simulink library "thc"  (R2021b)
settings: Solver=VariableStepAuto  StartTime=0.0  StopTime=10.0  RelTol=1e-3
undefined symbols (not defined in the file or in its folder): ATHC_APTCQA_X_C, ATHC_APTCQB_X_C, ATHC_dAy_X_C, ATHC_Qeq_X_kmh, ATHC_VbaseC_X_C, ATHC_VbaseC_Y_W, ATHC_VbaseD_X_C, ATHC_VbaseH_X_C, FALSE, KTHC_ACMaxMinT_sec, KTHC_aDeice_K, KTHC_AGSDefLv_K, KTHC_AGSLv1_K, KTHC_AGSLv2_K, KTHC_AGSLv3_K, KTHC_AGSLv4_K, KTHC_AGSLv5_K, KTHC_AirIntUpdateT_sec, KTHC_APTCOneZoneMax_W, KTHC_APTCPeriod_cnt, KTHC_APTCPWMEN_flg, KTHC_APTCQMaxC_W, KTHC_APTCQminC_W, KTHC_APTCQminD_W, KTHC_APTCQminRe1_W, KTHC_APTCQminRe_W, KTHC_APTCQoffT_cnt, KTHC_APTCQonT_cnt, KTHC_APTCRiLeMaxDff_W, KTHC_APTCRiLeMinDff_W, KTHC_BatInTempDef_C, KTHC_bDeice_K, KTHC_CompMaxDeice_rpm, KTHC_CompMinDeice_rpm, KTHC_CompSotxvOp_K, KTHC_CompSotxvOpLow_rpm, KTHC_CompSpdmax_rpm, KTHC_CompSpdmaxBC1_rpm, KTHC_CompSpdmaxBC_rpm, KTHC_CompSpdmid1_rpm, KTHC_CompSpdmid2_rpm, KTHC_CompSpdmid3_rpm, KTHC_CompSpdmid_rpm, KTHC_CompSpdmin_rpm, KTHC_DAPTCQ1_W, KTHC_DAPTCQ2_W, KTHC_DAPTCQ3_W, KTHC_DcChSetTemp_C, KTHC_DehumidityEN_flg, KTHC_DeiceCycTime_K, KTHC_DriveLevelWPTCBAH1_W, KTHC_DriveLevelWPTCBAH2_W, KTHC_DriveLevelWPTCBAH3_W, KTHC_DriveLevelWPTCBAH4_W, KTHC_DriveT1MinBAH_C, KTHC_DriveT2MaxBAH_C, KTHC_DriveT2MinBAH_C, KTHC_DriveT3MaxBAH_C, KTHC_DriveT3MinBAH_C, KTHC_DriveT4MaxBAH_C ... (+372)
libraries: simulink x140
(part 1 of 10)
settings Model: Creator=FVT20341  LastModifiedBy=FVT22063

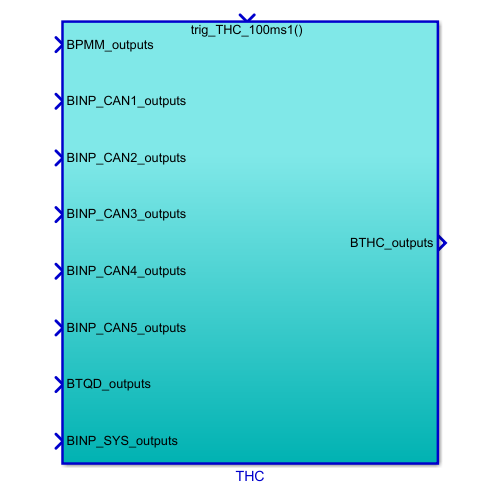
[thumbnail: Simulink's stored preview of the top-level diagram]
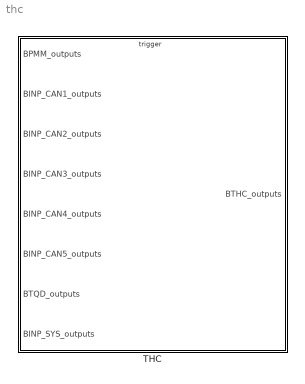
== system thc ==
  THC : Subsystem  TreatAsAtomicUnit=on
      settings: RTWSystemCode=Nonreusable function  RTWFcnNameOpts=Use subsystem name  RTWFileNameOpts=Use subsystem name

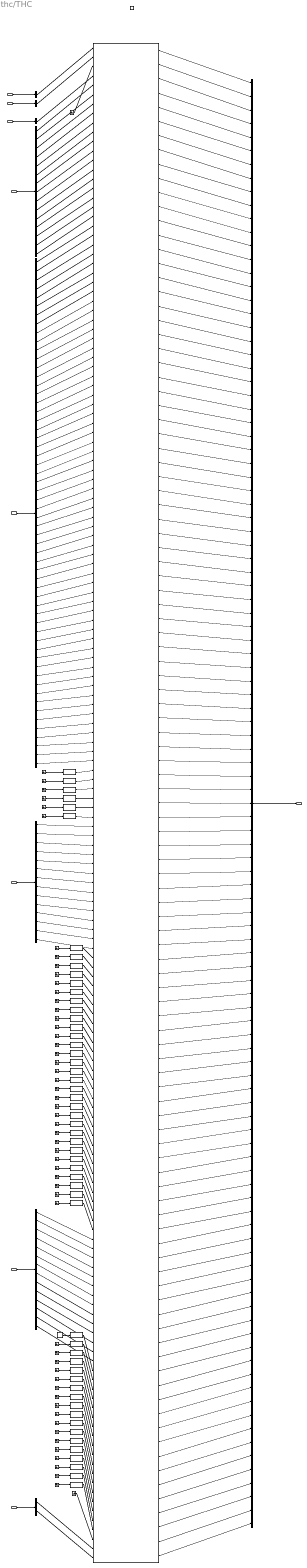
== system thc/THC ==
  BPMM_outputs : Inport  OutDataTypeStr=Bus: BPMM_outputs
  BINP_CAN1_outputs : Inport  Port=2  OutDataTypeStr=Bus: BINP_CAN1_outputs
  BINP_CAN2_outputs : Inport  Port=3  OutDataTypeStr=Bus: BINP_CAN2_outputs
  BINP_CAN3_outputs : Inport  Port=4  OutDataTypeStr=Bus: BINP_CAN3_outputs
  BINP_CAN4_outputs : Inport  Port=5  OutDataTypeStr=Bus: BINP_CAN4_outputs
  BINP_CAN5_outputs : Inport  Port=6  OutDataTypeStr=Bus: BINP_CAN5_outputs
  BTQD_outputs : Inport  Port=7  OutDataTypeStr=Bus: BTQD_outputs
  BINP_SYS_outputs : Inport  Port=8  OutDataTypeStr=Bus: BINP_SYS_outputs
  trig_THC_100ms1 : TriggerPort  TriggerType=function-call  VariantControl=(inherit)
  Bus Creator : BusCreator  Inputs=107  OutDataTypeStr=Bus: BTHC_outputs  NonVirtualBus=on
  Bus Selector : BusSelector  OutputSignals=VINP_FlashACModeMem_enum,VINP_FlashFace_flg,VINP_FlashFoot_flg,VINP_FlashFrost_flg,VINP_FlashFaceM_flg,VINP_FlashFootM_flg,VINP_FlashCCUSyncSts_flg,VINP_FlashACForceOFF_flg,VINP_FlashsigRecircSt_flg,VINP_FlashRecAutoFlg_flg,VINP_FlashAirIntenZone1M_enum,VINP_Flashfdefog_flg,VINP_FlashsigSetTempZon1St_C,VINP_FlashsigSetTempZon2StM_C
  Bus Selector1 : BusSelector  OutputSignals=VINP_VehSpeed_kph
  Bus Selector2 : BusSelector  OutputSignals=VINP_HVBMTempMax_C,VINP_HVBMTempMin_C,VINP_OBCTemp_C,VINP_DCDCTemp_C,VINP_RrTMTemp_C,VINP_RrMCUTemp_C,VINP_FrTMTemp_C,VINP_FrMCUTemp_C,VINP_ChrgPlugSta_enum,VINP_FrLLCTemp_C,VINP_RrLLCTemp_C,VINP_HVBIsoImpedenceN_Megaohm,VINP_HVBIsoImpedenceP_Megaohm,VINP_HVBHVILErr_flg,VINP_HVBattSOC_pct
  Bus Selector3 : BusSelector  OutputSignals=VINP_PTHighTact_C,VINP_COMPStatorSpd_rpm,VINP_CompProEN_flg,VINP_PTLowP1_KPa,VINP_PTLowT1_C,VINP_PTLowP2_KPa,VINP_PTLowT2_C,VINP_PTHighP_KPa,VINP_Tamb_C,VINP_BatInTemp_C,VINP_BatOutTemp_C,VINP_MotorInTemp_C,VINP_MotorOutTemp_C,VINP_Tincar_C,VINP_SolarL_W,VINP_SolarR_W,VINP_Tevap_C,VINP_TFaceL_C,VINP_TFaceR_C,VINP_TFootL_C,VINP_TFootR_C,VINP_TFootRr_C,VINP_TFaceRr_C,VINP_EACProtectEnable_enum,VINP_TambErr_enum,VINP_SolarLErr_enum,VINP_SolarRErr_enum,VINP_TevapErr_enum,VINP_TFaceLErr_enum,VINP_TFaceRErr_enum,VINP_TFootLErr_enum,VINP_TFootRErr_enum,VINP_TFaceRrErr_enum,VINP_TFootRrErr_enum,VINP_TincarErr_enum,VINP_BatInTempErr_enum,VINP_MotorInTempErr_enum,VINP_MotorOutTempErr_enum,VINP_FanErr_enum,VINP_AGSErr_enum,VINP_EWP3Err_enum,VINP_PTHighPErr_enum,VINP_PTHighTactErr_enum,VINP_SOV1Err_enum,VINP_SOV2Err_enum,VINP_SOV3Err_enum,VINP_EXV1Err_enum,VINP_EXV2Err_enum,VINP_COMPErr_enum,VINP_BlowerErr_enum,VINP_PTLowP1Err_enum,VINP_PTLowT1Err_enum,VINP_PTLowP2Err_enum,VINP_PTLowT2Err_enum,VINP_SOTXVErr_enum,VINP_FrntPTCRearLeActHeatPwr_W,VINP_FrntPTCRearRiActHeatPwr_W,VINP_FrntPTCRiActHeatPwr_W
  Bus Selector4 : BusSelector  OutputSignals=VINP_OFFACMODE_enum,VINP_FCPFrEvtBtnACMaxReq_flg,VINP_FCPFrEvtBtnACReq_flg,VINP_FCPFrEvtBtnAutoReq_flg,VINP_FCPFrEvtBtnSyncReq_flg,VINP_sigAirIntenZon1Req_enum,VINP_sigRecircReq_flg,VINP_sigFaceReq_flg,VINP_sigFootReq_flg,VINP_sigDfrstReq_flg,VINP_sigSetTempZon1Req_C,VINP_CANMsgValidIVI2_flg,VINP_sigSetTempZon2Req_C,VINP_SmartEcoModeSW_flg
  Bus Selector5 : BusSelector  OutputSignals=VTQD_ShiftGearPosn_enum
  Bus Selector6 : BusSelector  OutputSignals=VINP_RemoteACTemp_C,VINP_RemoteAutoReq_flg
  Bus Selector7 : BusSelector  OutputSignals=VPMM_PowerSta_enum
  Constant : Constant  Value=4
  Data Type Conversion{,1..4,6,8,10,12..35,48..50} (35 alike) : DataTypeConversion  OutDataTypeStr=uint8
  Data Type Conversion{5,7,9,11,36..47,55..57} (19 alike) : DataTypeConversion  OutDataTypeStr=boolean
  Ground{,1..19,25..26,28,37..54,56,58..70} (55 alike) : Ground
  ThermalControl : Subsystem
  BTHC_outputs : Outport  OutDataTypeStr=Bus: BTHC_outputs
  wires:
  BPMM_outputs/1 -> Bus Selector7/1
  Bus Selector7/1 -> ThermalControl/1(VPMM_PwrSta_enum)  "<VPMM_PowerSta_enum>"
  BINP_CAN1_outputs/1 -> Bus Selector1/1
  Bus Selector1/1 -> ThermalControl/4(VINP_VehSpeed_kph)  "<VINP_VehSpeed_kph>"
  BINP_CAN3_outputs/1 -> Bus Selector2/1
  Bus Selector2/3 -> ThermalControl/7(VINP_OBCTemp_C)  "<VINP_OBCTemp_C>"
  Bus Selector2/4 -> ThermalControl/8(VINP_DCDCTemp_C)  "<VINP_DCDCTemp_C>"
  Bus Selector2/2 -> ThermalControl/6(VINP_HVBMTempMin_C)  "<VINP_HVBMTempMin_C>"
  Bus Selector2/5 -> ThermalControl/9(VINP_RrTMTemp_C)  "<VINP_RrTMTemp_C>"
  Bus Selector2/1 -> ThermalControl/5(VINP_HVBMTempMax_C)  "<VINP_HVBMTempMax_C>"
  Bus Selector2/6 -> ThermalControl/10(VINP_RrMCUTemp_C)  "<VINP_RrMCUTemp_C>"
  Bus Selector2/7 -> ThermalControl/11(VINP_FrTMTemp_C)  "<VINP_FrTMTemp_C>"
  Bus Selector2/8 -> ThermalControl/12(VINP_FrMCUTemp_C)  "<VINP_FrMCUTemp_C>"
  ThermalControl/32(VTHC_sigClntTHvBattOut_C) -> Bus Creator/32  "VTHC_sigClntTHvBattOut_C"
  ThermalControl/31(VTHC_sigSetTempZon2St_C) -> Bus Creator/31  "VTHC_sigSetTempZon2St_C"
  ThermalControl/30(VTHC_sigSetTempZon1St_C) -> Bus Creator/30  "VTHC_sigSetTempZon1St_C"
  ThermalControl/29(VTHC_sigRecircSt_flg) -> Bus Creator/29  "VTHC_sigRecircSt_flg"
  ThermalControl/28(VTHC_sigWindDirZon1St_enum) -> Bus Creator/28  "VTHC_sigWindDirZon1St_enum"
  ThermalControl/27(VTHC_sigAirIntenZon1St_enum) -> Bus Creator/27  "VTHC_sigAirIntenZon1St_enum"
  ThermalControl/26(VTHC_CCUSyncLampSts_flg) -> Bus Creator/26  "VTHC_CCUSyncLampSts_flg"
  ThermalControl/25(VTHC_CCUACMaxLampSts_flg) -> Bus Creator/25  "VTHC_CCUACMaxLampSts_flg"
  ThermalControl/24(VTHC_CCUAutoLampSts_flg) -> Bus Creator/24  "VTHC_CCUAutoLampSts_flg"
  ThermalControl/23(VTHC_CCUACLampSts_flg) -> Bus Creator/23  "VTHC_CCUACLampSts_flg"
  ThermalControl/22(VTHC_CabinMode_enum) -> Bus Creator/22  "VTHC_CabinMode_enum"
  ThermalControl/21(VTHC_EDriveMode_enum) -> Bus Creator/21  "VTHC_EDriveMode_enum"
  ThermalControl/20(VTHC_BatteryMode_enum) -> Bus Creator/20  "VTHC_BatteryMode_enum"
  ThermalControl/19(VTHC_FDBlowerCmd_pct) -> Bus Creator/19  "VTHC_FDBlowerCmd_pct"
  ThermalControl/17(VTHC_FDFrRiAPTCHeatPwrCmd_W) -> Bus Creator/17  "VTHC_FDFrRiAPTCHeatPwrCmd_W"
  ThermalControl/18(VTHC_FDRrAPTCHeatPwrCmd_W) -> Bus Creator/18  "VTHC_FDRrAPTCHeatPwrCmd_W"
  ThermalControl/16(VTHC_FDFrLeAPTCHeatPwrCmd_W) -> Bus Creator/16  "VTHC_FDFrLeAPTCHeatPwrCmd_W"
  ThermalControl/15(VTHC_FDEWP3Cmd_enum) -> Bus Creator/15  "VTHC_FDEWP3Cmd_enum"
  ThermalControl/14(VTHC_FDEWP2Cmd_enum) -> Bus Creator/14  "VTHC_FDEWP2Cmd_enum"
  ThermalControl/13(VTHC_FDEWP1Cmd_enum) -> Bus Creator/13  "VTHC_FDEWP1Cmd_enum"
  ThermalControl/12(VTHC_FDAGSCmd_enum) -> Bus Creator/12  "VTHC_FDAGSCmd_enum"
  ThermalControl/11(VTHC_CoolgFanActDuty_pct) -> Bus Creator/11  "VTHC_CoolgFanActDuty_pct"
  ThermalControl/10(VTHC_FDFrWPTCHeatPwrCmd_W) -> Bus Creator/10  "VTHC_FDFrWPTCHeatPwrCmd_W"
  ThermalControl/9(VTHC_FDTWVCmd_pct) -> Bus Creator/9  "VTHC_FDTWVCmd_pct"
  ThermalControl/8(VTHC_FDFWVCmd_flg) -> Bus Creator/8  "VTHC_FDFWVCmd_flg"
  ThermalControl/7(VTHC_FDSOTXVCmd_flg) -> Bus Creator/7  "VTHC_FDSOTXVCmd_flg"
  ThermalControl/6(VTHC_FDEXV2Cmd_step) -> Bus Creator/6  "VTHC_FDEXV2Cmd_step"
  ThermalControl/5(VTHC_FDEXV1Cmd_step) -> Bus Creator/5  "VTHC_FDEXV1Cmd_step"
  ThermalControl/4(VTHC_FDSOV3Cmd_flg) -> Bus Creator/4  "VTHC_FDSOV3Cmd_flg"
  ThermalControl/3(VTHC_FDSOV2Cmd_flg) -> Bus Creator/3  "VTHC_FDSOV2Cmd_flg"
  ThermalControl/2(VTHC_FDSOV1Cmd_flg) -> Bus Creator/2  "VTHC_FDSOV1Cmd_flg"
  ThermalControl/1(VTHC_FDCompCmd_rpm) -> Bus Creator/1  "VTHC_FDCompCmd_rpm"
  Bus Creator/1 -> BTHC_outputs/1  "BTHC_outputs"
  BINP_CAN4_outputs/1 -> Bus Selector3/1  "BINP_CAN4_outputs"
  Bus Selector3/4 -> ThermalControl/23(VINP_PTLowP1_kPa)  "<VINP_PTLowP1_KPa>"
  Bus Selector3/5 -> ThermalControl/24(VINP_PTLowT1_C)  "<VINP_PTLowT1_C>"
  Bus Selector3/6 -> ThermalControl/25(VINP_PTLowP2_kPa)  "<VINP_PTLowP2_KPa>"
  Bus Selector3/7 -> ThermalControl/26(VINP_PTLowT2_C)  "<VINP_PTLowT2_C>"
  Bus Selector3/8 -> ThermalControl/27(VINP_PTHighP_kPa)  "<VINP_PTHighP_KPa>"
  Bus Selector3/9 -> ThermalControl/28(VINP_Tamb_C)  "<VINP_Tamb_C>"
  Bus Selector3/10 -> ThermalControl/29(VINP_BatInTemp_C)  "<VINP_BatInTemp_C>"
  Bus Selector3/11 -> ThermalControl/30(VINP_BatOutTemp_C)  "<VINP_BatOutTemp_C>"
  Bus Selector3/12 -> ThermalControl/31(VINP_MotorInTemp_C)  "<VINP_MotorInTemp_C>"
  Bus Selector3/13 -> ThermalControl/32(VINP_MotorOutTemp_C)  "<VINP_MotorOutTemp_C>"
  Bus Selector3/14 -> ThermalControl/33(VINP_Tincar_C)  "<VINP_Tincar_C>"
  Bus Selector3/15 -> ThermalControl/34(VINP_SolarL_W)  "<VINP_SolarL_W>"
  Bus Selector3/16 -> ThermalControl/35(VINP_SolarR_W)  "<VINP_SolarR_W>"
  Bus Selector3/17 -> ThermalControl/36(VINP_Tevap_C)  "<VINP_Tevap_C>"
  Bus Selector3/18 -> ThermalControl/37(VINP_TFaceL_C)  "<VINP_TFaceL_C>"
  Bus Selector3/19 -> ThermalControl/38(VINP_TFaceR_C)  "<VINP_TFaceR_C>"
  Bus Selector3/20 -> ThermalControl/39(VINP_TFootL_C)  "<VINP_TFootL_C>"
  Bus Selector3/21 -> ThermalControl/40(VINP_TFootR_C)  "<VINP_TFootR_C>"
  Bus Selector3/22 -> ThermalControl/41(VINP_TFootRr_C)  "<VINP_TFootRr_C>"
  Bus Selector3/23 -> ThermalControl/42(VINP_TFaceRr_C)  "<VINP_TFaceRr_C>"
  BINP_CAN2_outputs/1 -> Bus Selector4/1  "BINP_CAN2_outputs"
  Bus Selector4/2 -> ThermalControl/85(VINP_FCPFrEvtBtnACMaxReq_flg)  "<VINP_FCPFrEvtBtnACMaxReq_flg>"
  Bus Selector4/3 -> ThermalControl/86(VINP_FCPFrEvtBtnACReq_flg)  "<VINP_FCPFrEvtBtnACReq_flg>"
  Bus Selector4/4 -> ThermalControl/87(VINP_FCPFrEvtBtnAutoReq_flg)  "<VINP_FCPFrEvtBtnAutoReq_flg>"
  Bus Selector4/5 -> ThermalControl/88(VINP_FCPFrEvtBtnSyncReq_flg)  "<VINP_FCPFrEvtBtnSyncReq_flg>"
  Bus Selector4/6 -> ThermalControl/89(VINP_sigAirIntenZon1Req_enum)  "<VINP_sigAirIntenZon1Req_enum>"
  Bus Selector4/7 -> ThermalControl/90(VINP_sigRecircReq_flg)  "<VINP_sigRecircReq_flg>"
  Bus Selector4/8 -> ThermalControl/91(VINP_sigFaceReq_flg)  "<VINP_sigFaceReq_flg>"
  Bus Selector4/9 -> ThermalControl/92(VINP_sigFootReq_flg)  "<VINP_sigFootReq_flg>"
  Bus Selector4/10 -> ThermalControl/93(VINP_sigFrostReq_flg)  "<VINP_sigDfrstReq_flg>"
  Bus Selector4/11 -> ThermalControl/94(VINP_sigSetTempZon1Req_C)  "<VINP_sigSetTempZon1Req_C>"
  Bus Selector4/12 -> ThermalControl/95(VINP_CANMsgValidIVI2_flg)  "<VINP_CANMsgValidIVI2_flg>"
  Bus Selector4/13 -> ThermalControl/96(VINP_sigSetTempZon2Req_C)  "<VINP_sigSetTempZon2Req_C>"
  Bus Selector2/9 -> ThermalControl/13(VINP_ChrgPlugSta_enum)  "<VINP_ChrgPlugSta_enum>"
  Bus Selector3/2 -> ThermalControl/21(VINP_COMP_StatorSpd_RPM)  "<VINP_COMPStatorSpd_rpm>"
  Bus Selector3/3 -> ThermalControl/22(VINP_CompProEN_flg)  "<VINP_CompProEN_flg>"
  ThermalControl/33(VTHC_sigCbnSolarLeft_W) -> Bus Creator/33  "VTHC_sigCbnSolarLeft_W"
  ThermalControl/34(VTHC_sigClntTHvBattIn_C) -> Bus Creator/34  "VTHC_sigClntTHvBattIn_C"
  ThermalControl/35(VTHC_sigCbnSolarRight_W) -> Bus Creator/35  "VTHC_sigCbnSolarRight_W"
  ThermalControl/36(VTHC_sigAmbAirT_C) -> Bus Creator/36  "VTHC_sigAmbAirT_C"
  ThermalControl/37(VTHC_sigCbnAirT_C) -> Bus Creator/37  "VTHC_sigCbnAirT_C"
  ThermalControl/38(VTHC_ACSubMode_enum) -> Bus Creator/38  "VTHC_ACSubMode_enum"
  ThermalControl/40(VTHC_CompP_K) -> Bus Creator/40  "VTHC_CompP_K"
  ThermalControl/41(VTHC_CompI_K) -> Bus Creator/41  "VTHC_CompI_K"
  ThermalControl/42(VTHC_CompU_K) -> Bus Creator/42  "VTHC_CompU_K"
  ThermalControl/43(VTHC_CompDeltaU_K) -> Bus Creator/43  "VTHC_CompDeltaU_K"
  ThermalControl/44(VTHC_Compe_K) -> Bus Creator/44  "VTHC_Compe_K"
  ThermalControl/45(VTHC_Blowere_K) -> Bus Creator/45  "VTHC_Blowere_K"
  ThermalControl/46(VTHC_BlowerP_K) -> Bus Creator/46  "VTHC_BlowerP_K"
  ThermalControl/47(VTHC_BlowerU_K) -> Bus Creator/47  "VTHC_BlowerU_K"
  ThermalControl/48(VTHC_Vbase_pct) -> Bus Creator/48  "VTHC_Vbase_pct"
  ThermalControl/49(VTHC_BlowerI_K) -> Bus Creator/49  "VTHC_BlowerI_K"
  ThermalControl/50(VTHC_EXV2P_K) -> Bus Creator/50  "VTHC_EXV2P_K"
  ThermalControl/51(VTHC_EXV2I_K) -> Bus Creator/51  "VTHC_EXV2I_K"
  ThermalControl/52(VTHC_EXV2U_K) -> Bus Creator/52  "VTHC_EXV2U_K"
  ThermalControl/53(VTHC_EXV2e_K) -> Bus Creator/53  "VTHC_EXV2e_K"
  ThermalControl/54(VTHC_APTCP_K) -> Bus Creator/54  "VTHC_APTCP_K"
  ThermalControl/55(VTHC_APTCI_K) -> Bus Creator/55  "VTHC_APTCI_K"
  ThermalControl/56(VTHC_APTCU_K) -> Bus Creator/56  "VTHC_APTCU_K"
  ThermalControl/57(VTHC_APTCe_K) -> Bus Creator/57  "VTHC_APTCe_K"
  ThermalControl/58(VTHC_EXV1P_K) -> Bus Creator/58  "VTHC_EXV1P_K"
  ThermalControl/59(VTHC_EXV1I_K) -> Bus Creator/59  "VTHC_EXV1I_K"
  ThermalControl/60(VTHC_EXV1U_K) -> Bus Creator/60  "VTHC_EXV1U_K"
  ThermalControl/61(VTHC_EXV1e_K) -> Bus Creator/61  "VTHC_EXV1e_K"
  BTQD_outputs/1 -> Bus Selector5/1
  Bus Selector5/1 -> ThermalControl/2(VTQD_ShiftGearPosn_enum)  "<VTQD_ShiftGearPosn_enum>"
  Bus Selector3/1 -> ThermalControl/20(VINP_PTHighTact_C)  "<VINP_PTHighTact_C>"
  Bus Selector2/10 -> ThermalControl/14(VINP_FrLLCTemp_C)  "<VINP_FrLLCTemp_C>"
  Bus Selector2/11 -> ThermalControl/15(VINP_RrLLCTemp_C)  "<VINP_RrLLCTemp_C>"
  Ground/1 -> ThermalControl/3(VSCP_AGSCloseSta_flg)
  Bus Selector4/1 -> ThermalControl/84(VINP_OFFACMODE_enum)  "<VINP_OFFACMODE_enum>"
  ThermalControl/39(VTHC_FDRecyAutoCmd_enum) -> Bus Creator/39  "VTHC_FDRecyAutoCmd_enum"
  Bus Selector3/24 -> ThermalControl/43(VINP_EACProtectEnable_enum)  "<VINP_EACProtectEnable_enum>"
  Bus Selector3/25 -> ThermalControl/44(Tamb_Err)  "<VINP_TambErr_enum>"
  Bus Selector3/26 -> ThermalControl/45(SolarL_Err)  "<VINP_SolarLErr_enum>"
  Bus Selector3/27 -> ThermalControl/46(SolarR_Err)  "<VINP_SolarRErr_enum>"
  Bus Selector3/28 -> ThermalControl/47(Tevap_Err)  "<VINP_TevapErr_enum>"
  Bus Selector3/29 -> ThermalControl/48(T_Face_L_Err)  "<VINP_TFaceLErr_enum>"
  Bus Selector3/30 -> ThermalControl/49(T_Face_R_Err)  "<VINP_TFaceRErr_enum>"
  Bus Selector3/31 -> ThermalControl/50(T_Foot_L_Err)  "<VINP_TFootLErr_enum>"
  Bus Selector3/32 -> ThermalControl/51(T_Foot_R_Err)  "<VINP_TFootRErr_enum>"
  Bus Selector3/33 -> ThermalControl/52(T_Face_Rr_Err)  "<VINP_TFaceRrErr_enum>"
  Bus Selector3/34 -> ThermalControl/53(T_Foot_Rr_Err)  "<VINP_TFootRrErr_enum>"
  Bus Selector3/35 -> ThermalControl/54(Tincar_Err)  "<VINP_TincarErr_enum>"
  Bus Selector3/36 -> ThermalControl/55(Bat_In_Temp_Err)  "<VINP_BatInTempErr_enum>"
  Bus Selector3/37 -> ThermalControl/56(Motor_In_Temp_Err)  "<VINP_MotorInTempErr_enum>"
  Bus Selector3/38 -> ThermalControl/57(Motor_Out_Temp_Err)  "<VINP_MotorOutTempErr_enum>"
  Bus Selector3/39 -> ThermalControl/58(Fan_Err)  "<VINP_FanErr_enum>"
  Bus Selector3/40 -> ThermalControl/59(AGS_Err)  "<VINP_AGSErr_enum>"
  Bus Selector3/41 -> ThermalControl/60(EWP3_Err)  "<VINP_EWP3Err_enum>"
  Bus Selector3/42 -> ThermalControl/61(PT_High_P_Err)  "<VINP_PTHighPErr_enum>"
  Bus Selector3/43 -> ThermalControl/62(PT_High_Tact_Err)  "<VINP_PTHighTactErr_enum>"
  Bus Selector3/44 -> ThermalControl/63(SOV1_Err)  "<VINP_SOV1Err_enum>"
  Bus Selector3/45 -> ThermalControl/64(SOV2_Err)  "<VINP_SOV2Err_enum>"
  Bus Selector3/46 -> ThermalControl/65(SOV3_Err)  "<VINP_SOV3Err_enum>"
  Bus Selector3/47 -> ThermalControl/66(EXV1_Err)  "<VINP_EXV1Err_enum>"
  Bus Selector3/48 -> ThermalControl/67(EXV2_Err)  "<VINP_EXV2Err_enum>"
  Bus Selector3/49 -> ThermalControl/68(Comp_Err)  "<VINP_COMPErr_enum>"
  Bus Selector3/50 -> ThermalControl/69(Blower_Err)  "<VINP_BlowerErr_enum>"
  Bus Selector3/51 -> ThermalControl/70(PT_Low_P1_Err)  "<VINP_PTLowP1Err_enum>"
  Bus Selector3/52 -> ThermalControl/71(PT_Low_T1_Err)  "<VINP_PTLowT1Err_enum>"
  Bus Selector3/53 -> ThermalControl/72(PT_Low_P2_Err)  "<VINP_PTLowP2Err_enum>"
  Bus Selector3/54 -> ThermalControl/73(PT_Low_T2_Err)  "<VINP_PTLowT2Err_enum>"
  Bus Selector3/55 -> ThermalControl/74(SOTXV_Err)  "<VINP_SOTXVErr_enum>"
  ThermalControl/62(VTHC_ACModeMem_enum) -> Bus Creator/62  "VTHC_ACModeMem_enum"
  ThermalControl/63(VTHC_Face_flg) -> Bus Creator/63  "VTHC_Face_flg"
  ThermalControl/64(VTHC_Foot_flg) -> Bus Creator/64  "VTHC_Foot_flg"
  ThermalControl/65(VTHC_Frost_flg) -> Bus Creator/65  "VTHC_Frost_flg"
  ThermalControl/66(VTHC_FaceM_flg) -> Bus Creator/66  "VTHC_FaceM_flg"
  ThermalControl/67(VTHC_FootM_flg) -> Bus Creator/67  "VTHC_FootM_flg"
  ThermalControl/68(VTHC_CCUSyncSts_flg) -> Bus Creator/68  "VTHC_CCUSyncSts_flg"
  ThermalControl/69(VTHC_ACForceOFF_flg) -> Bus Creator/69  "VTHC_ACForceOFF_flg"
  ThermalControl/70(VTHC_RecAutoFlg_flg) -> Bus Creator/70  "VTHC_RecAutoFlg_flg"
  ThermalControl/71(VTHC_AirIntenZone1M_enum) -> Bus Creator/71  "VTHC_AirIntenZone1M_enum"
  ThermalControl/72(VTHC_fdefog_flg) -> Bus Creator/72  "VTHC_fdefog_flg"
  BINP_SYS_outputs/1 -> Bus Selector/1  "BINP_SYS_output"
  Bus Selector/3 -> ThermalControl/130(EEP_Foot)  "<VINP_FlashFoot_flg>"
  Bus Selector/2 -> ThermalControl/129(EEP_Face)  "<VINP_FlashFace_flg>"
  Bus Selector/4 -> ThermalControl/131(EEP_Frost)  "<VINP_FlashFrost_flg>"
  Bus Selector/1 -> ThermalControl/128(EEP_ACModeMem)  "<VINP_FlashACModeMem_enum>"
  Bus Selector/5 -> ThermalControl/132(EEP_FaceM)  "<VINP_FlashFaceM_flg>"
  Bus Selector/6 -> ThermalControl/133(EEP_FootM)  "<VINP_FlashFootM_flg>"
  Bus Selector/7 -> ThermalControl/134(EEP_CCUSyncSts)  "<VINP_FlashCCUSyncSts_flg>"
  Bus Selector/8 -> ThermalControl/135(EEP_ACForceOFF)  "<VINP_FlashACForceOFF_flg>"
  Bus Selector/9 -> ThermalControl/136(EEP_sigRecircSt)  "<VINP_FlashsigRecircSt_flg>"
  Bus Selector/10 -> ThermalControl/137(EEP_RecAutoFlg)  "<VINP_FlashRecAutoFlg_flg>"
  Bus Selector/11 -> ThermalControl/138(EEP_AirIntenZone1iM)  "<VINP_FlashAirIntenZone1M_enum>"
  Bus Selector/12 -> ThermalControl/139(EEP_fdefog)  "<VINP_Flashfdefog_flg>"
  ThermalControl/73(VTHC_sigSetTempZon2StM_C) -> Bus Creator/73
  Bus Selector/13 -> ThermalControl/140(EEP_sigSetTempZon1St)  "<VINP_FlashsigSetTempZon1St_C>"
  Bus Selector/14 -> ThermalControl/141(EEP_sigSetTempZon2StM)  "<VINP_FlashsigSetTempZon2StM_C>"
  BINP_CAN5_outputs/1 -> Bus Selector6/1
  Bus Selector6/2 -> ThermalControl/162(VINP_RemoteAutoReq_flg)  "<VINP_RemoteAutoReq_flg>"
  Bus Selector6/1 -> ThermalControl/161(VINP_RemoteACTemp_C)  "<VINP_RemoteACTemp_C>"
  Bus Selector4/14 -> ThermalControl/97(VINP_SmartEcoModeSW_flg)  "<VINP_SmartEcoModeSW_flg>"
  Bus Selector2/12 -> ThermalControl/16(VINP_HVBIsoImpedenceN_Mohm)  "<VINP_HVBIsoImpedenceN_Megaohm>"
  Bus Selector2/13 -> ThermalControl/17(VINP_HVBIsoImpedenceP_Mohm)  "<VINP_HVBIsoImpedenceP_Megaohm>"
  Bus Selector2/14 -> ThermalControl/18(VINP_HVBHVILErr_flg)  "<VINP_HVBHVILErr_flg>"
  Bus Selector3/56 -> ThermalControl/75(VINP_FrntPTCRearLeActHeatPwr_W)  "<VINP_FrntPTCRearLeActHeatPwr_W>"
  Bus Selector3/57 -> ThermalControl/76(VINP_FrntPTCRearRiActHeatPwr_W)  "<VINP_FrntPTCRearRiActHeatPwr_W>"
  Bus Selector3/58 -> ThermalControl/77(VINP_FrntPTCRiActHeatPwr_W)  "<VINP_FrntPTCRiActHeatPwr_W>"
  ThermalControl/74(VTHC_sigDfrstSt_flg) -> Bus Creator/74
  ThermalControl/75(VTHC_FDCTHCAirIntZ3Sta_enum) -> Bus Creator/75
  ThermalControl/76(VTHC_FDCTHCDrEVentModeSta_enum) -> Bus Creator/76
  ThermalControl/77(VTHC_FDCTHCPsEVentModeSta_enum) -> Bus Creator/77
  ThermalControl/78(VTHC_FDCTHCDrEVentZSta_enum) -> Bus Creator/78
  ThermalControl/79(VTHC_FDCTHCCLEVentZSta_enum) -> Bus Creator/79
  ThermalControl/80(VTHC_FDCTHCPsEVentZSta_enum) -> Bus Creator/80
  ThermalControl/81(VTHC_FDCTHCCREVentZSta_enum) -> Bus Creator/81
  ThermalControl/82(VTHC_FDCTHCDrEVentYSta_enum) -> Bus Creator/82
  ThermalControl/83(VTHC_FDCTHCDrVentENSta_flg) -> Bus Creator/83
  ThermalControl/84(VTHC_FDCTHCCLEVentYSta_enum) -> Bus Creator/84
  ThermalControl/85(VTHC_FDCTHCCLVentENSta_flg) -> Bus Creator/85
  ThermalControl/86(VTHC_FDCTHCPsEVentYSta_enum) -> Bus Creator/86
  ThermalControl/87(VTHC_FDCTHCPsVentENSta_flg) -> Bus Creator/87
  ThermalControl/88(VTHC_FDCTHCCREVentYSta_enum) -> Bus Creator/88
  ThermalControl/89(VTHC_FDCTHCCRVentENSta_flg) -> Bus Creator/89
  Ground44/1 -> ThermalControl/160(APTCFailDTC)
  ThermalControl/90(VTHC_FDCTHCMAPTCForceOFFSta_flg) -> Bus Creator/90
  ThermalControl/91(VTHC_DrVentEN_flg) -> Bus Creator/91
  ThermalControl/92(VTHC_CLVentEN_flg) -> Bus Creator/92
  ThermalControl/93(VTHC_PsVentEN_flg) -> Bus Creator/93
  ThermalControl/94(VTHC_CRVentEN_flg) -> Bus Creator/94
  ThermalControl/95(VTHC_Z1TUP_flg) -> Bus Creator/95
  ThermalControl/96(VTHC_Z1TDN_flg) -> Bus Creator/96
  ThermalControl/97(VTHC_Z2TUP_flg) -> Bus Creator/97
  ThermalControl/98(VTHC_Z2TDN_flg) -> Bus Creator/98
  ThermalControl/99(VTHC_FDCFGSAirIntSta_enum) -> Bus Creator/99
  ThermalControl/100(VTHC_FDCFGSChSta_enum) -> Bus Creator/100
  ThermalControl/101(VTHC_FDCFGSAirIntCmd_enum) -> Bus Creator/101
  ThermalControl/102(VTHC_FDCFGSFuncSta_flg) -> Bus Creator/102
  ThermalControl/103(VTHC_FDCFGSChCmd_enum) -> Bus Creator/103
  ThermalControl/104(VTHC_FDCFGSIONSWSta_flg) -> Bus Creator/104
  ThermalControl/105(VTHC_FDCFGSIONCmd_flg) -> Bus Creator/105
  ThermalControl/106(VTHC_FDCFGSLearnCmd_enum) -> Bus Creator/106
  Bus Selector2/15 -> ThermalControl/19(VINP_HVBattSOC_pct)  "<VINP_HVBattSOC_pct>"
  ThermalControl/107(VTHC_FDCTHCMPreWPTCHeatSta_enum) -> Bus Creator/107
  Ground3/1 -> Data Type Conversion/1
  Data Type Conversion/1 -> ThermalControl/83(VINP_FGSMotorInitSta_enum)
  Ground54/1 -> Data Type Conversion2/1
  Data Type Conversion1/1 -> ThermalControl/142(EEP_FDCTHCAirIntZ3Sta)
  Constant/1 -> Data Type Conversion1/1
  Data Type Conversion2/1 -> ThermalControl/158(FGSChStaM)
  Ground37/1 -> Data Type Conversion3/1
  Ground38/1 -> Data Type Conversion5/1
  Ground39/1 -> Data Type Conversion4/1
  Ground42/1 -> Data Type Conversion8/1
  Ground41/1 -> Data Type Conversion9/1
  Ground40/1 -> Data Type Conversion7/1
  Ground43/1 -> Data Type Conversion6/1
  Ground48/1 -> Data Type Conversion10/1
  Ground45/1 -> Data Type Conversion11/1
  Ground46/1 -> Data Type Conversion13/1
  Ground47/1 -> Data Type Conversion12/1
  Ground51/1 -> Data Type Conversion16/1
  Ground50/1 -> Data Type Conversion17/1
  Ground49/1 -> Data Type Conversion15/1
  Ground52/1 -> Data Type Conversion14/1
  Data Type Conversion17/1 -> ThermalControl/143(VINP_FDCTHCPsEVentModeStaM_enum)
  Data Type Conversion16/1 -> ThermalControl/144(VINP_FDCTHCDrEVentModeStaM_enum)
  Data Type Conversion15/1 -> ThermalControl/145(VINP_FDCTHCDrEVentZStaM_enum)
  Data Type Conversion14/1 -> ThermalControl/146(VINP_FDCTHCCLEVentZStaM_enum)
  Data Type Conversion13/1 -> ThermalControl/147(VINP_FDCTHCPsEVentZStaM_enum)
  Data Type Conversion12/1 -> ThermalControl/148(VINP_FDCTHCCREVentZStaM_enum)
  Data Type Conversion11/1 -> ThermalControl/149(EEP_DrVentENM)
  Data Type Conversion10/1 -> ThermalControl/150(VINP_FDCTHCDrEVentYStaM_enum)
  Data Type Conversion9/1 -> ThermalControl/151(EEP_CLVentENM)
  Data Type Conversion8/1 -> ThermalControl/152(VINP_FDCTHCCLEVentYStaM_enum)
  Data Type Conversion7/1 -> ThermalControl/153(EEP_PsVentENM)
  Data Type Conversion6/1 -> ThermalControl/154(VINP_FDCTHCPsEVentYStaM_enum)
  Data Type Conversion5/1 -> ThermalControl/155(EEP_CRVentENM)
  Data Type Conversion4/1 -> ThermalControl/156(VINP_FDCTHCCREVentYStaM_enum)
  Data Type Conversion3/1 -> ThermalControl/157(FGSAirIntStaM)
  Ground53/1 -> Data Type Conversion18/1
  Data Type Conversion18/1 -> ThermalControl/159("IONSWStaM ")
  Ground70/1 -> Data Type Conversion27/1
  Ground69/1 -> Data Type Conversion23/1
  Ground66/1 -> Data Type Conversion24/1
  Ground67/1 -> Data Type Conversion26/1
  Ground68/1 -> Data Type Conversion25/1
  Ground64/1 -> Data Type Conversion21/1
  Ground63/1 -> Data Type Conversion22/1
  Ground62/1 -> Data Type Conversion20/1
  Ground65/1 -> Data Type Conversion19/1
  Ground61/1 -> Data Type Conversion32/1
  Ground58/1 -> Data Type Conversion33/1
  Ground59/1 -> Data Type Conversion35/1
  Ground60/1 -> Data Type Conversion34/1
  Ground56/1 -> Data Type Conversion31/1
  Data Type Conversion26/1 -> ThermalControl/111(VINP_IVIDrBlowerModeSta_enum)
  Data Type Conversion25/1 -> ThermalControl/112(VINP_IVIPsBlowerModeSta_enum)
  Data Type Conversion24/1 -> ThermalControl/113(VINP_IVIDrBlowerZSta_enum)
  Data Type Conversion23/1 -> ThermalControl/114(VINP_IVICLBlowerZSta_enum)
  Data Type Conversion22/1 -> ThermalControl/115(VINP_IVIPsBlowerZSta_enum)
  Data Type Conversion21/1 -> ThermalControl/116(VINP_IVICRBlowerZSta_enum)
  Data Type Conversion20/1 -> ThermalControl/117(VINP_IVIDrBlowerYSta_enum)
  Data Type Conversion19/1 -> ThermalControl/118(VINP_IVICLBlowerYSta_enum)
  Data Type Conversion35/1 -> ThermalControl/119(VINP_IVIPsBlowerYSta_enum)
  Data Type Conversion34/1 -> ThermalControl/120(VINP_IVICRBlowerYSta_enum)
  Data Type Conversion33/1 -> ThermalControl/121(VINP_IVIsigScreenReq_Sta)
  Data Type Conversion32/1 -> ThermalControl/122(VINP_IVIFGSAirIntCmd_enum)
  Data Type Conversion31/1 -> ThermalControl/123(VINP_IVIFGSChCmd_enum)
  Data Type Conversion27/1 -> ThermalControl/127(ECOSW)
  Ground8/1 -> Data Type Conversion48/1
  Ground19/1 -> Data Type Conversion43/1
  Data Type Conversion43/1 -> ThermalControl/98(VINP_HMIACBtnCmd_flg)
  Data Type Conversion48/1 -> ThermalControl/110(VINP_IVIAirIntZ3Cmd_enum)
  Ground1/1 -> Data Type Conversion36/1
  Ground9/1 -> Data Type Conversion37/1
  Ground10/1 -> Data Type Conversion38/1
  Ground12/1 -> Data Type Conversion41/1
  Ground14/1 -> Data Type Conversion40/1
  Ground11/1 -> Data Type Conversion39/1
  Ground13/1 -> Data Type Conversion42/1
  Ground17/1 -> Data Type Conversion47/1
  Ground15/1 -> Data Type Conversion44/1
  Ground18/1 -> Data Type Conversion45/1
  Ground16/1 -> Data Type Conversion46/1
  Data Type Conversion36/1 -> ThermalControl/99(VINP_HMIACAutoBtnCmd_flg)
  Data Type Conversion38/1 -> ThermalControl/100(VINP_HMIACRecycleBtnCmd_flg)
  Data Type Conversion37/1 -> ThermalControl/101(VINP_HMIACFrDefogBtnCmd_flg)
  Data Type Conversion42/1 -> ThermalControl/102(VINP_HMIZ1SetTPCmd_flg)
  Data Type Conversion39/1 -> ThermalControl/103(VINP_HMIZ1SetTMCmd_flg)
  Data Type Conversion41/1 -> ThermalControl/104(VINP_HMIZ2SetTPCmd_flg)
  Data Type Conversion40/1 -> ThermalControl/105(VINP_HMIZ2SetTMCmd_flg)
  Data Type Conversion47/1 -> ThermalControl/106(VINP_HMIACWindDirPCmd_flg)
  Data Type Conversion44/1 -> ThermalControl/107(VINP_HMIACWindDirMCmd_flg)
  Data Type Conversion46/1 -> ThermalControl/108(VINP_HMIACAirIntPCmd_flg)
  Data Type Conversion45/1 -> ThermalControl/109(VINP_HMIACAirIntDirMCmd_flg)
  Ground26/1 -> Data Type Conversion57/1
  Ground28/1 -> Data Type Conversion56/1
  Ground25/1 -> Data Type Conversion55/1
  Data Type Conversion55/1 -> ThermalControl/124(VINP_IVIIONSWCmd_flg)
  Data Type Conversion57/1 -> ThermalControl/125(VINP_IVIWPTCSWSta_flg)
  Data Type Conversion56/1 -> ThermalControl/126(VINP_IVIZon1WindDirSWReqSta_flg)
  Ground2/1 -> Data Type Conversion28/1
  Ground4/1 -> Data Type Conversion30/1
  Ground5/1 -> Data Type Conversion29/1
  Ground7/1 -> Data Type Conversion49/1
  Ground6/1 -> Data Type Conversion50/1
  Data Type Conversion50/1 -> ThermalControl/78(VINP_ZFRTHCDrEVentActYSta_enum)
  Data Type Conversion49/1 -> ThermalControl/79(VINP_ZFRTHCCLEVentActYSta_enum)
  Data Type Conversion30/1 -> ThermalControl/80(VINP_ZFRTHCPsEVentActYSta_enum)
  Data Type Conversion29/1 -> ThermalControl/81(VINP_ZFRTHCCREVentActYSta_enum)
  Data Type Conversion28/1 -> ThermalControl/82(VINP_FGSAirIntSta_enum)
